simulink library "iWalkerLib"  (R2014a)
settings: Solver=ode45  StartTime=0.0  StopTime=10.0  RelTol=1e-3
undefined symbols (not defined in the file): fclose, fread, fwrite, iWheelServer, laserServer, socket
settings Model: Creator=Brian  LastModifiedBy=Brian

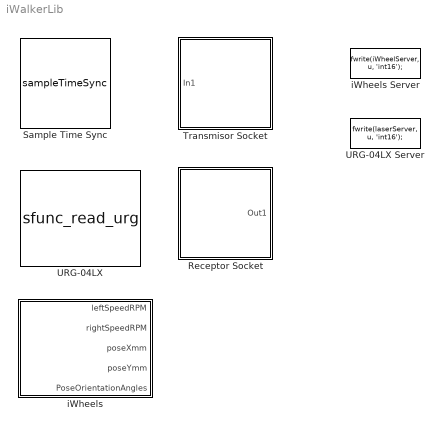
== system iWalkerLib ==
  Receptor Socket : Subsystem  InitFcn=|  mask(Server Socket){ip='0.0.0.0', port=4000, SampleTime=1}
      | % Obtenemos parametros de la Mask
      | block = gcb;
      | ip = get_param(block, 'ip');
      | port = str2num(get_param(block, 'port'));
      | Tsocket = get_param(block, 'SampleTime');
      | 
      | % Configuramos el sample time
      | set_param([block], 'SampleTime', Tsocket);
      | 
      | % Creamos el socket y lo configuramos
      | disp('Opening socket...');
      | disp(ip)
      | disp(port)
      | disp(Tsocket)
      | x = 'hello';
      | disp(x)
      | %socket = tcpip(ip, port, 'NetworkRole', 'client');
      | socket = tcpip('localhost', port, 'NetworkRole', 'client');
      | set(socket, 'InputBufferSize', 4000);
      | set(socket, 'ByteOrder', 'littleEndian');
      | set(socket, 'Timeout', 10000);
      | fopen(socket);
      | 
      | 
      | clear block ip port
      mask prompts: ip "IP adress"; SampleTime "Sample Time"
      mask help:
      | TCP/IP communication block.
      | To accept any client, the IP  may be set to the wild card address
      | of '0.0.0.0'.
      settings: DeleteFcn=|
      | fclose(socket);
      | 
      | clear socket
      mask Display:
      | image('router.png');
      | port_label('output', 1, 'Rx');
  Sample Time Sync : S-Function  Priority=8  FunctionName=sampleTimeSync  EnableBusSupport=off
      mask Display: image('timeSetup.png')
  Transmisor Socket : Subsystem  InitFcn=|  mask(Client Network Socket){ip='localhost', port=4000}
      | % Obtenemos parametros de la Mask
      | block = gcb;
      | ip = get_param(block, 'ip');
      | port = str2num(get_param(block, 'port'));
      | 
      | % Creamos el socket y lo configuramos
      | disp('Opening socket...');
      | socket = tcpip(ip, port, 'NetworkRole', 'client');
      | set(socket, 'OutputBufferSize', 4000);
      | set(t, 'ByteOrder', 'littleEndian');
      | fopen(socket);
      | 
      | clear block ip port
      mask prompts: ip "IP adress"
      mask help:
      | TCP/IP communication block.
      | The IP and Port parameters are from the server.
      settings: DeleteFcn=|
      | fclose(socket);
      | 
      | clear socket
      mask Display:
      | image('router.png');
      | port_label('input', 1, 'Tx');
  URG-04LX : S-Function  FunctionName=sfunc_read_urg  EnableBusSupport=off  mask{COM=1, SampleTime=0.5, Verbose=off}
      mask prompts: SampleTime "Sample time"
      mask Display:
      | image('urg_top.jpg')
      | port_label('output', 1, 'Range');
  URG-04LX Server : MATLABFcn  InitFcn=|  StopFcn=fclose(laserServer);  MATLABFcn=fwrite(laserServer, u, 'int16');  OutputDimensions=0  mask{port=4001}
      | port = str2num(get_param(gcb, 'port'));
      | laserServer = tcpip('0.0.0.0', port, 'NetworkRole', 'server');
      | set(laserServer, 'OutputBufferSize', 15000);
      | fopen(laserServer);
  iWheels : Subsystem
      mask Display:
      | image('iWheel.jpg')
      | port_label('output', 1, 'left rpm')
      | port_label('output', 2, 'right rpm')
      | port_label('output', 3, 'x mm')
      | port_label('output', 4, 'y mm')
      | port_label('output', 5, 'theta º')
  iWheels Server : MATLABFcn  InitFcn=|  StopFcn=fclose(iWheelServer);  MATLABFcn=fwrite(iWheelServer, u, 'int16');  OutputDimensions=0  mask{port=4000}
      | port = str2num(get_param(gcb, 'port'));
      | iWheelServer = tcpip('0.0.0.0', port, 'NetworkRole', 'server');
      | fopen(iWheelServer);

== system iWalkerLib/Receptor Socket ==
  Interpreted MATLAB Function : MATLABFcn  MATLABFcn=fread(u, 1, 'int16')
  Out1 : Outport
  wires:
  Interpreted MATLAB Function/1 -> Out1/1

== system iWalkerLib/Transmisor Socket ==
  In1 : Inport
  Interpreted MATLAB Function : MATLABFcn  MATLABFcn=fwrite(socket, u, 'int16')  OutputDimensions=0
  wires:
  In1/1 -> Interpreted MATLAB Function/1

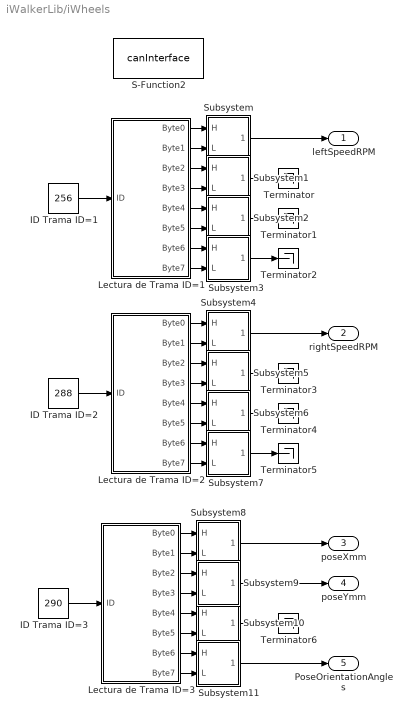
== system iWalkerLib/iWheels ==
  ID Trama ID=1 : Constant  Priority=-1  Value=256
  ID Trama ID=2 : Constant  Priority=-1  Value=288
  ID Trama ID=3 : Constant  Priority=-1  Value=290
  Lectura de Trama ID=1 : Subsystem  Priority=0
  Lectura de Trama ID=2 : Subsystem  Priority=0
  Lectura de Trama ID=3 : Subsystem  Priority=0
  S-Function2 : S-Function  Priority=-1  FunctionName=canInterface  EnableBusSupport=off
  Subsystem : Subsystem
  Subsystem1 : Subsystem
  Subsystem10 : Subsystem
  Subsystem11 : Subsystem
  Subsystem2 : Subsystem
  Subsystem3 : Subsystem
  Subsystem4 : Subsystem
  Subsystem5 : Subsystem
  Subsystem6 : Subsystem
  Subsystem7 : Subsystem
  Subsystem8 : Subsystem
  Subsystem9 : Subsystem
  Terminator{,1..6} (7 alike) : Terminator
  leftSpeedRPM : Outport
  rightSpeedRPM : Outport  Port=2
  poseXmm : Outport  Port=3
  poseYmm : Outport  Port=4
  PoseOrientationAngles : Outport  Port=5
  wires:
  Subsystem11/1(Out1) -> PoseOrientationAngles/1
  Subsystem10/1(Out1) -> Terminator6/1
  Subsystem9/1(Out1) -> poseYmm/1
  Subsystem8/1(Out1) -> poseXmm/1
  Subsystem4/1(Out1) -> rightSpeedRPM/1
  Subsystem/1(Out1) -> leftSpeedRPM/1
  ID Trama ID=3/1 -> Lectura de Trama ID=3/1(ID)
  Lectura de Trama ID=3/1(Byte0) -> Subsystem8/1(H)
  Lectura de Trama ID=3/2(Byte1) -> Subsystem8/2(L)
  Lectura de Trama ID=3/3(Byte2) -> Subsystem9/1(H)
  Lectura de Trama ID=3/4(Byte3) -> Subsystem9/2(L)
  Lectura de Trama ID=3/5(Byte4) -> Subsystem10/1(H)
  Lectura de Trama ID=3/6(Byte5) -> Subsystem10/2(L)
  Lectura de Trama ID=3/7(Byte6) -> Subsystem11/1(H)
  Lectura de Trama ID=3/8(Byte7) -> Subsystem11/2(L)
  Subsystem5/1(Out1) -> Terminator3/1
  Subsystem6/1(Out1) -> Terminator4/1
  Subsystem7/1(Out1) -> Terminator5/1
  ID Trama ID=2/1 -> Lectura de Trama ID=2/1(ID)
  Lectura de Trama ID=2/1(Byte0) -> Subsystem4/1(H)
  Lectura de Trama ID=2/2(Byte1) -> Subsystem4/2(L)
  Lectura de Trama ID=2/3(Byte2) -> Subsystem5/1(H)
  Lectura de Trama ID=2/4(Byte3) -> Subsystem5/2(L)
  Lectura de Trama ID=2/5(Byte4) -> Subsystem6/1(H)
  Lectura de Trama ID=2/6(Byte5) -> Subsystem6/2(L)
  Lectura de Trama ID=2/7(Byte6) -> Subsystem7/1(H)
  Lectura de Trama ID=2/8(Byte7) -> Subsystem7/2(L)
  ID Trama ID=1/1 -> Lectura de Trama ID=1/1(ID)
  Lectura de Trama ID=1/1(Byte0) -> Subsystem/1(H)
  Lectura de Trama ID=1/2(Byte1) -> Subsystem/2(L)
  Lectura de Trama ID=1/3(Byte2) -> Subsystem1/1(H)
  Lectura de Trama ID=1/4(Byte3) -> Subsystem1/2(L)
  Subsystem1/1(Out1) -> Terminator/1
  Lectura de Trama ID=1/5(Byte4) -> Subsystem2/1(H)
  Lectura de Trama ID=1/6(Byte5) -> Subsystem2/2(L)
  Subsystem2/1(Out1) -> Terminator1/1
  Lectura de Trama ID=1/7(Byte6) -> Subsystem3/1(H)
  Lectura de Trama ID=1/8(Byte7) -> Subsystem3/2(L)
  Subsystem3/1(Out1) -> Terminator2/1

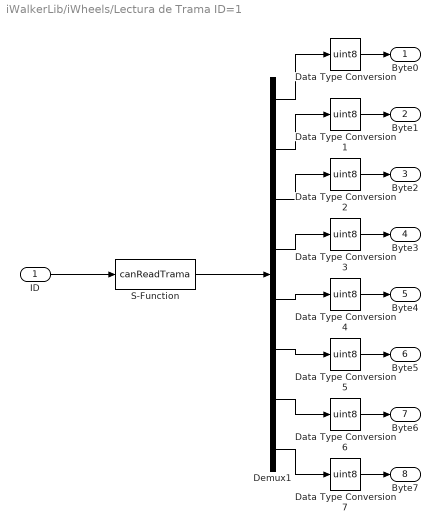
== system iWalkerLib/iWheels/Lectura de Trama ID=1 ==
  ID : Inport
  Data Type Conversion{,1..7} (8 alike) : DataTypeConversion  OutDataTypeStr=uint8  ConvertRealWorld=Stored Integer (SI)
  Demux1 : Demux  Outputs=8
  S-Function : S-Function  Priority=0  FunctionName=canReadTrama  EnableBusSupport=off
  Byte0 : Outport
  Byte1 : Outport  Port=2
  Byte2 : Outport  Port=3
  Byte3 : Outport  Port=4
  Byte4 : Outport  Port=5
  Byte5 : Outport  Port=6
  Byte6 : Outport  Port=7
  Byte7 : Outport  Port=8
  wires:
  Data Type Conversion3/1 -> Byte3/1
  Data Type Conversion2/1 -> Byte2/1
  Demux1/8 -> Data Type Conversion7/1
  Demux1/7 -> Data Type Conversion6/1
  Demux1/6 -> Data Type Conversion5/1
  Demux1/5 -> Data Type Conversion4/1
  Demux1/4 -> Data Type Conversion3/1
  Demux1/3 -> Data Type Conversion2/1
  Demux1/2 -> Data Type Conversion1/1
  Demux1/1 -> Data Type Conversion/1
  Data Type Conversion/1 -> Byte0/1
  Data Type Conversion1/1 -> Byte1/1
  Data Type Conversion4/1 -> Byte4/1
  Data Type Conversion5/1 -> Byte5/1
  Data Type Conversion6/1 -> Byte6/1
  Data Type Conversion7/1 -> Byte7/1
  S-Function/1 -> Demux1/1
  ID/1 -> S-Function/1

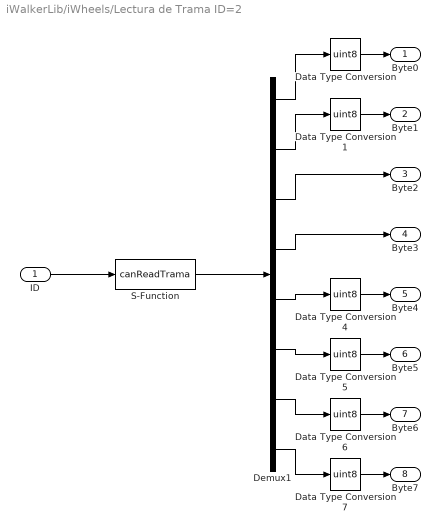
== system iWalkerLib/iWheels/Lectura de Trama ID=2 ==
  ID : Inport
  Data Type Conversion{,1,4..7} (6 alike) : DataTypeConversion  OutDataTypeStr=uint8  ConvertRealWorld=Stored Integer (SI)
  Demux1 : Demux  Outputs=8
  S-Function : S-Function  Priority=0  FunctionName=canReadTrama  EnableBusSupport=off
  Byte0 : Outport
  Byte1 : Outport  Port=2
  Byte2 : Outport  Port=3
  Byte3 : Outport  Port=4
  Byte4 : Outport  Port=5
  Byte5 : Outport  Port=6
  Byte6 : Outport  Port=7
  Byte7 : Outport  Port=8
  wires:
  Demux1/8 -> Data Type Conversion7/1
  Demux1/7 -> Data Type Conversion6/1
  Demux1/6 -> Data Type Conversion5/1
  Demux1/5 -> Data Type Conversion4/1
  Demux1/4 -> Byte3/1
  Demux1/3 -> Byte2/1
  Demux1/2 -> Data Type Conversion1/1
  Demux1/1 -> Data Type Conversion/1
  Data Type Conversion/1 -> Byte0/1
  Data Type Conversion1/1 -> Byte1/1
  Data Type Conversion4/1 -> Byte4/1
  Data Type Conversion5/1 -> Byte5/1
  Data Type Conversion6/1 -> Byte6/1
  Data Type Conversion7/1 -> Byte7/1
  S-Function/1 -> Demux1/1
  ID/1 -> S-Function/1

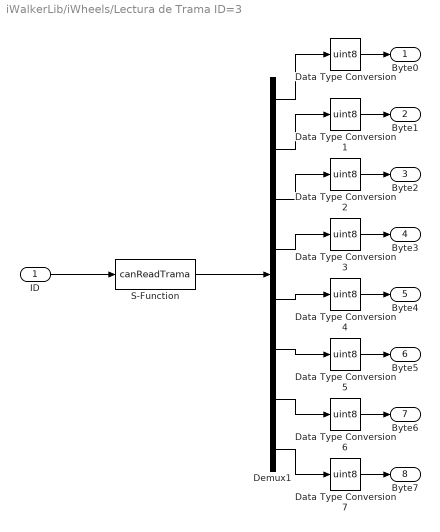
== system iWalkerLib/iWheels/Lectura de Trama ID=3 ==
  ID : Inport
  Data Type Conversion{,1..7} (8 alike) : DataTypeConversion  OutDataTypeStr=uint8  ConvertRealWorld=Stored Integer (SI)
  Demux1 : Demux  Outputs=8
  S-Function : S-Function  Priority=0  FunctionName=canReadTrama  EnableBusSupport=off
  Byte0 : Outport
  Byte1 : Outport  Port=2
  Byte2 : Outport  Port=3
  Byte3 : Outport  Port=4
  Byte4 : Outport  Port=5
  Byte5 : Outport  Port=6
  Byte6 : Outport  Port=7
  Byte7 : Outport  Port=8
  wires:
  Data Type Conversion3/1 -> Byte3/1
  Data Type Conversion2/1 -> Byte2/1
  Demux1/8 -> Data Type Conversion7/1
  Demux1/7 -> Data Type Conversion6/1
  Demux1/6 -> Data Type Conversion5/1
  Demux1/5 -> Data Type Conversion4/1
  Demux1/4 -> Data Type Conversion3/1
  Demux1/3 -> Data Type Conversion2/1
  Demux1/2 -> Data Type Conversion1/1
  Demux1/1 -> Data Type Conversion/1
  Data Type Conversion/1 -> Byte0/1
  Data Type Conversion1/1 -> Byte1/1
  Data Type Conversion4/1 -> Byte4/1
  Data Type Conversion5/1 -> Byte5/1
  Data Type Conversion6/1 -> Byte6/1
  Data Type Conversion7/1 -> Byte7/1
  S-Function/1 -> Demux1/1
  ID/1 -> S-Function/1

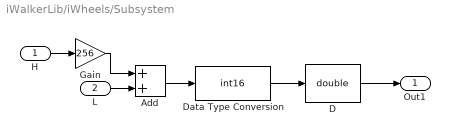
== system iWalkerLib/iWheels/Subsystem ==
  H : Inport
  L : Inport  Port=2
  Add : Sum
  D : DataTypeConversion  OutDataTypeStr=double  ConvertRealWorld=Stored Integer (SI)
  Data Type Conversion : DataTypeConversion  OutDataTypeStr=int16
  Gain : Gain  Gain=256
  Out1 : Outport
  wires:
  D/1 -> Out1/1
  Data Type Conversion/1 -> D/1
  Add/1 -> Data Type Conversion/1
  L/1 -> Add/2
  H/1 -> Gain/1
  Gain/1 -> Add/1

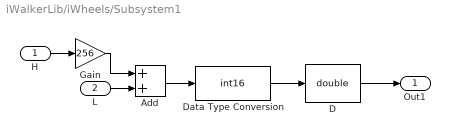
== system iWalkerLib/iWheels/Subsystem1 ==
  H : Inport
  L : Inport  Port=2
  Add : Sum
  D : DataTypeConversion  OutDataTypeStr=double  ConvertRealWorld=Stored Integer (SI)
  Data Type Conversion : DataTypeConversion  OutDataTypeStr=int16
  Gain : Gain  Gain=256
  Out1 : Outport
  wires:
  Gain/1 -> Add/1
  H/1 -> Gain/1
  L/1 -> Add/2
  Add/1 -> Data Type Conversion/1
  Data Type Conversion/1 -> D/1
  D/1 -> Out1/1

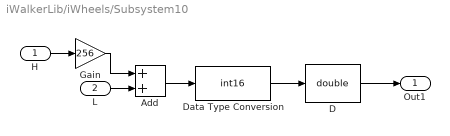
== system iWalkerLib/iWheels/Subsystem10 ==
  H : Inport
  L : Inport  Port=2
  Add : Sum
  D : DataTypeConversion  OutDataTypeStr=double  ConvertRealWorld=Stored Integer (SI)
  Data Type Conversion : DataTypeConversion  OutDataTypeStr=int16
  Gain : Gain  Gain=256
  Out1 : Outport
  wires:
  D/1 -> Out1/1
  Data Type Conversion/1 -> D/1
  Add/1 -> Data Type Conversion/1
  L/1 -> Add/2
  H/1 -> Gain/1
  Gain/1 -> Add/1

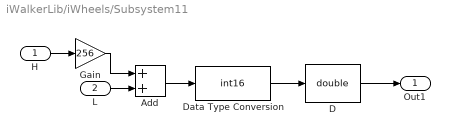
== system iWalkerLib/iWheels/Subsystem11 ==
  H : Inport
  L : Inport  Port=2
  Add : Sum
  D : DataTypeConversion  OutDataTypeStr=double  ConvertRealWorld=Stored Integer (SI)
  Data Type Conversion : DataTypeConversion  OutDataTypeStr=int16
  Gain : Gain  Gain=256
  Out1 : Outport
  wires:
  Gain/1 -> Add/1
  H/1 -> Gain/1
  L/1 -> Add/2
  Add/1 -> Data Type Conversion/1
  Data Type Conversion/1 -> D/1
  D/1 -> Out1/1

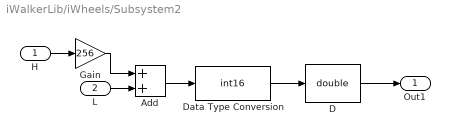
== system iWalkerLib/iWheels/Subsystem2 ==
  H : Inport
  L : Inport  Port=2
  Add : Sum
  D : DataTypeConversion  OutDataTypeStr=double  ConvertRealWorld=Stored Integer (SI)
  Data Type Conversion : DataTypeConversion  OutDataTypeStr=int16
  Gain : Gain  Gain=256
  Out1 : Outport
  wires:
  D/1 -> Out1/1
  Data Type Conversion/1 -> D/1
  Add/1 -> Data Type Conversion/1
  L/1 -> Add/2
  H/1 -> Gain/1
  Gain/1 -> Add/1

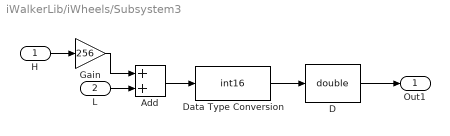
== system iWalkerLib/iWheels/Subsystem3 ==
  H : Inport
  L : Inport  Port=2
  Add : Sum
  D : DataTypeConversion  OutDataTypeStr=double  ConvertRealWorld=Stored Integer (SI)
  Data Type Conversion : DataTypeConversion  OutDataTypeStr=int16
  Gain : Gain  Gain=256
  Out1 : Outport
  wires:
  Gain/1 -> Add/1
  H/1 -> Gain/1
  L/1 -> Add/2
  Add/1 -> Data Type Conversion/1
  Data Type Conversion/1 -> D/1
  D/1 -> Out1/1

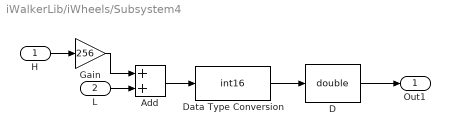
== system iWalkerLib/iWheels/Subsystem4 ==
  H : Inport
  L : Inport  Port=2
  Add : Sum
  D : DataTypeConversion  OutDataTypeStr=double  ConvertRealWorld=Stored Integer (SI)
  Data Type Conversion : DataTypeConversion  OutDataTypeStr=int16
  Gain : Gain  Gain=256
  Out1 : Outport
  wires:
  D/1 -> Out1/1
  Data Type Conversion/1 -> D/1
  Add/1 -> Data Type Conversion/1
  L/1 -> Add/2
  H/1 -> Gain/1
  Gain/1 -> Add/1

== system iWalkerLib/iWheels/Subsystem5 ==
  H : Inport
  L : Inport  Port=2
  Add : Sum
  D : DataTypeConversion  OutDataTypeStr=double  ConvertRealWorld=Stored Integer (SI)
  Data Type Conversion : DataTypeConversion  OutDataTypeStr=int16
  Gain : Gain  Gain=256
  Out1 : Outport
  wires:
  Gain/1 -> Add/1
  H/1 -> Gain/1
  L/1 -> Add/2
  Add/1 -> Data Type Conversion/1
  Data Type Conversion/1 -> D/1
  D/1 -> Out1/1

== system iWalkerLib/iWheels/Subsystem6 ==
  H : Inport
  L : Inport  Port=2
  Add : Sum
  D : DataTypeConversion  OutDataTypeStr=double  ConvertRealWorld=Stored Integer (SI)
  Data Type Conversion : DataTypeConversion  OutDataTypeStr=int16
  Gain : Gain  Gain=256
  Out1 : Outport
  wires:
  D/1 -> Out1/1
  Data Type Conversion/1 -> D/1
  Add/1 -> Data Type Conversion/1
  L/1 -> Add/2
  H/1 -> Gain/1
  Gain/1 -> Add/1

== system iWalkerLib/iWheels/Subsystem7 ==
  H : Inport
  L : Inport  Port=2
  Add : Sum
  D : DataTypeConversion  OutDataTypeStr=double  ConvertRealWorld=Stored Integer (SI)
  Data Type Conversion : DataTypeConversion  OutDataTypeStr=int16
  Gain : Gain  Gain=256
  Out1 : Outport
  wires:
  Gain/1 -> Add/1
  H/1 -> Gain/1
  L/1 -> Add/2
  Add/1 -> Data Type Conversion/1
  Data Type Conversion/1 -> D/1
  D/1 -> Out1/1

== system iWalkerLib/iWheels/Subsystem8 ==
  H : Inport
  L : Inport  Port=2
  Add : Sum
  D : DataTypeConversion  OutDataTypeStr=double  ConvertRealWorld=Stored Integer (SI)
  Data Type Conversion : DataTypeConversion  OutDataTypeStr=int16
  Gain : Gain  Gain=256
  Out1 : Outport
  wires:
  D/1 -> Out1/1
  Data Type Conversion/1 -> D/1
  Add/1 -> Data Type Conversion/1
  L/1 -> Add/2
  H/1 -> Gain/1
  Gain/1 -> Add/1

== system iWalkerLib/iWheels/Subsystem9 ==
  H : Inport
  L : Inport  Port=2
  Add : Sum
  D : DataTypeConversion  OutDataTypeStr=double  ConvertRealWorld=Stored Integer (SI)
  Data Type Conversion : DataTypeConversion  OutDataTypeStr=int16
  Gain : Gain  Gain=256
  Out1 : Outport
  wires:
  Gain/1 -> Add/1
  H/1 -> Gain/1
  L/1 -> Add/2
  Add/1 -> Data Type Conversion/1
  Data Type Conversion/1 -> D/1
  D/1 -> Out1/1
